simulink model "hdl_model_fixed"  (R2024a)
settings: Solver=FixedStepDiscrete  StartTime=0.0  StopTime=SIM_TIME  RelTol=1e-3
model workspace (MAT data in the model file):
  HDLVAXIManagerConfig = hdlverifier.internal.AXIMaster.ConfigParams
undefined symbols (not defined in the file or in its folder): BUFFER_LEN, SAMPLING_FREQ, signal_1
libraries: hdlsllib x4, simulink x1, dspsrcs4 x1, simulink_extras x1, dsphdlxfrm2 x1
settings Model: DataTypeOverride=Off  SimulationMode=accelerator  Creator=Jan Rosa  LastModifiedBy=Jan Rosa
settings OptimizationCC: BlockReduction=off  ConditionallyExecuteInputs=off  DefaultParameterBehavior=Inlined  InheritOutputTypeSmallerThanSingle=on
settings DebuggingCC: SignalRangeChecking=warning  AlgebraicLoopMsg=error  SolverPrmCheckMsg=warning  SingleTaskRateTransMsg=error  UnderSpecifiedDataTypeMsg=warning  UnconnectedInputMsg=error  UnconnectedOutputMsg=error  UnconnectedLineMsg=error  ModelReferenceVersionMismatchMessage=warning  ModelReferenceIOMismatchMessage=warning  ModelReferenceNoExplicitFinalValueMsg=warning  StateNameClashWarn=warning
settings HardwareCC: ProdBitPerPointer=32  ProdBitPerSizeT=32  ProdBitPerPtrDiffT=32  ProdLargestAtomicFloat=None  ProdIntDivRoundTo=Undefined  ProdEndianess=Unspecified  ProdWordSize=32  ProdHWDeviceType=ASIC/FPGA->ASIC/FPGA  TargetBitPerPointer=64  TargetBitPerSizeT=64  TargetBitPerPtrDiffT=64  TargetLongLongMode=on  TargetIntDivRoundTo=Zero  TargetEndianess=LittleEndian  TargetWordSize=64  TargetHWDeviceType=Custom Processor->MATLAB Host Computer  ProdEqTarget=off
settings ModelReferenceCC: EnableRefExpFcnMdlSchedulingChecks=on  EnableParallelModelReferenceBuilds=on

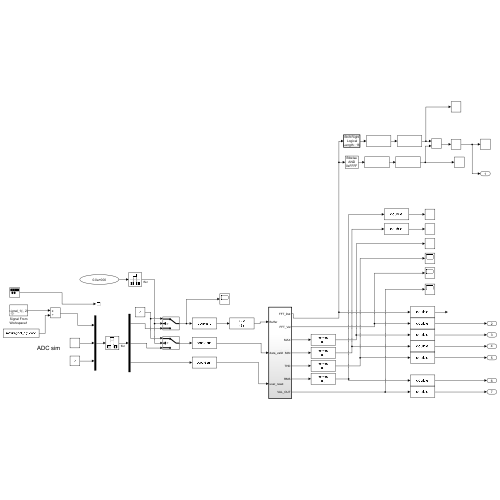
[thumbnail: Simulink's stored preview of the top-level diagram]
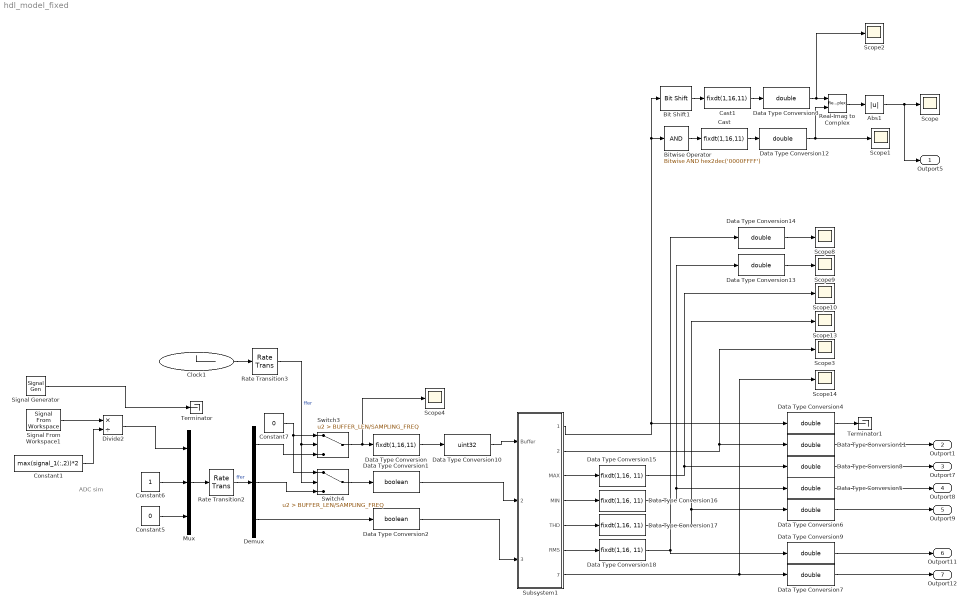
== system hdl_model_fixed ==
  note: ADC sim
  Abs1 : Abs  SaturateOnIntegerOverflow=off
  Bit Shift1 : hdlsllib/Logic and Bit Operations/Bit Shift  mode=Shift Right Logical  N=16
  Bitwise Operator : simulink/Logic and Bit Operations/Bitwise Operator  logicop=AND  UseBitMask=on  BitMask=hex2dec('0000FFFF')  BitMaskRealWorld=Stored Integer
  Cast : DataTypeConversion  OutDataTypeStr=fixdt(1,16,11)  ConvertRealWorld=Stored Integer (SI)  SaturateOnIntegerOverflow=off  RndMeth=Floor
  Cast1 : DataTypeConversion  OutDataTypeStr=fixdt(1,16,11)  ConvertRealWorld=Stored Integer (SI)  SaturateOnIntegerOverflow=off  RndMeth=Floor
  Clock1 : Clock
  Constant1 : Constant  Value=max(signal_1(:,2))*2
  Constant5 : Constant  Value=0
  Constant6 : Constant
  Constant7 : Constant  Value=0  SampleTime=1/SAMPLING_FREQ
  Data Type Conversion : DataTypeConversion  OutDataTypeStr=fixdt(1,16,11)  SaturateOnIntegerOverflow=off  RndMeth=Floor  LockScale=on
  Data Type Conversion1 : DataTypeConversion  OutDataTypeStr=boolean  SaturateOnIntegerOverflow=off  RndMeth=Floor  LockScale=on
  Data Type Conversion10 : DataTypeConversion  OutDataTypeStr=uint32  ConvertRealWorld=Stored Integer (SI)  SaturateOnIntegerOverflow=off  RndMeth=Floor
  Data Type Conversion{3..9,11..14} (11 alike) : DataTypeConversion  OutDataTypeStr=double  SaturateOnIntegerOverflow=off  RndMeth=Floor
  Data Type Conversion{15..18} (4 alike) : DataTypeConversion  OutDataTypeStr=fixdt(1,16, 11)  ConvertRealWorld=Stored Integer (SI)  SaturateOnIntegerOverflow=off  RndMeth=Floor
  Data Type Conversion2 : DataTypeConversion  OutDataTypeStr=boolean  SaturateOnIntegerOverflow=off  RndMeth=Floor  LockScale=on
  Demux : Demux  Outputs=3
  Divide2 : Product  Inputs=*/
  Mux : Mux  Inputs=3
  Rate Transition2 : RateTransition  Integrity=off  Deterministic=off  OutPortSampleTime=1/SAMPLING_FREQ
  Rate Transition3 : RateTransition  Integrity=off  Deterministic=off  OutPortSampleTime=1/SAMPLING_FREQ
  Real-Imag to Complex : RealImagToComplex
  Scope{,1..4,8..10,13..14} (10 alike) : Scope
  Signal Generator : SignalGenerator  WaveForm=square  Amplitude=1/2.001  Frequency=SAMPLING_FREQ/(16*16)
  Signal From Workspace1 : dspsrcs4/Signal From Workspace  X=signal_1(:, 2)  Ts=1.28/SAMPLING_FREQ  nsamps=1  OutputAfterFinalValue=Cyclic repetition  ignoreOrWarnInputAndFrameLengths=off  OutputFrames=off
  Subsystem1 : Subsystem  TreatAsAtomicUnit=on
  Switch3 : Switch  Criteria=u2 > Threshold  Threshold=BUFFER_LEN/SAMPLING_FREQ  SaturateOnIntegerOverflow=off  InputSameDT=off
  Switch4 : Switch  Criteria=u2 > Threshold  Threshold=BUFFER_LEN/SAMPLING_FREQ  SaturateOnIntegerOverflow=off  InputSameDT=off
  Terminator : Terminator
  Terminator1 : Terminator
  Outport5 : Outport
  Outport1 : Outport  Port=2
  Outport7 : Outport  Port=3
  Outport8 : Outport  Port=4
  Outport9 : Outport  Port=5
  Outport11 : Outport  Port=6
  Outport12 : Outport  Port=7
  wires:
  Subsystem1/1(FFT_Dat) -> Data Type Conversion4/1, Bitwise Operator/1, Bit Shift1/1
  Constant7/1 -> Switch4/1, Switch3/1
  Rate Transition3/1 -> Switch4/2, Switch3/2  "ffer"
  Subsystem1/7(VAL_OUT) -> Data Type Conversion7/1, Scope14/1
  Subsystem1/3(MAX) -> Data Type Conversion15/1
  Demux/2 -> Switch4/3
  Clock1/1 -> Rate Transition3/1
  Demux/3 -> Data Type Conversion2/1
  Subsystem1/5(THD) -> Data Type Conversion17/1
  Switch3/1 -> Scope4/1, Data Type Conversion/1
  Demux/1 -> Switch3/3
  Mux/1 -> Rate Transition2/1
  Subsystem1/4(MIN) -> Data Type Conversion16/1
  Abs1/1 -> Outport5/1, Scope/1
  Rate Transition2/1 -> Demux/1  "ffer"
  Constant5/1 -> Mux/3
  Signal From Workspace1/1 -> Divide2/1
  Constant6/1 -> Mux/2
  Constant1/1 -> Divide2/2
  Subsystem1/6(RMS) -> Data Type Conversion18/1
  Data Type Conversion8/1 -> Outport7/1
  Data Type Conversion5/1 -> Outport8/1
  Data Type Conversion6/1 -> Outport9/1
  Data Type Conversion7/1 -> Outport12/1
  Data Type Conversion9/1 -> Outport11/1
  Data Type Conversion11/1 -> Outport1/1
  Data Type Conversion3/1 -> Scope2/1, Real-Imag to Complex/1
  Real-Imag to Complex/1 -> Abs1/1
  Bit Shift1/1 -> Cast1/1
  Bitwise Operator/1 -> Cast/1
  Data Type Conversion12/1 -> Scope1/1, Real-Imag to Complex/2
  Cast/1 -> Data Type Conversion12/1
  Cast1/1 -> Data Type Conversion3/1
  Data Type Conversion14/1 -> Scope8/1
  Data Type Conversion13/1 -> Scope9/1
  Switch4/1 -> Data Type Conversion1/1
  Data Type Conversion2/1 -> Subsystem1/3(user_reset)
  Data Type Conversion1/1 -> Subsystem1/2(data_valid)
  Data Type Conversion/1 -> Data Type Conversion10/1
  Subsystem1/2(FFT_Val) -> Scope3/1, Data Type Conversion11/1
  Data Type Conversion10/1 -> Subsystem1/1(Buffer)
  Data Type Conversion15/1 -> Data Type Conversion8/1, Scope10/1
  Data Type Conversion16/1 -> Data Type Conversion5/1, Data Type Conversion13/1
  Data Type Conversion17/1 -> Data Type Conversion6/1, Scope13/1
  Data Type Conversion18/1 -> Data Type Conversion9/1, Data Type Conversion14/1
  Data Type Conversion4/1 -> Terminator1/1
  Signal Generator/1 -> Terminator/1
  Divide2/1 -> Mux/1

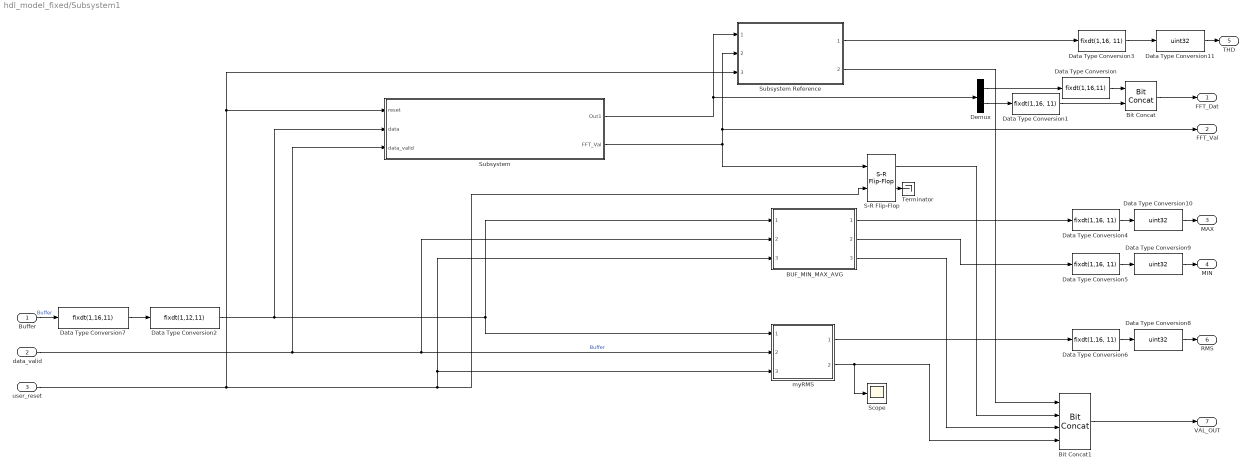
== system hdl_model_fixed/Subsystem1 ==
  Buffer : Inport  OutDataTypeStr=uint32
  data_valid : Inport  Port=2
  user_reset : Inport  Port=3
  BUF_MIN_MAX_AVG : Subsystem  TreatAsAtomicUnit=on  ReferencedSubsystem=BUF_MIN_MAX_AVG_fixed
  Bit Concat : hdlsllib/Logic and Bit Operations/Bit Concat  numInputs=2
  Bit Concat1 : hdlsllib/Logic and Bit Operations/Bit Concat  numInputs=4
  Data Type Conversion : DataTypeConversion  OutDataTypeStr=fixdt(1,16,11)  SaturateOnIntegerOverflow=off  RndMeth=Floor
  Data Type Conversion{1,3..6} (5 alike) : DataTypeConversion  OutDataTypeStr=fixdt(1,16, 11)  SaturateOnIntegerOverflow=off  RndMeth=Floor
  Data Type Conversion{8..11} (4 alike) : DataTypeConversion  OutDataTypeStr=uint32  ConvertRealWorld=Stored Integer (SI)  SaturateOnIntegerOverflow=off  RndMeth=Floor
  Data Type Conversion2 : DataTypeConversion  OutDataTypeStr=fixdt(1,12,11)  SaturateOnIntegerOverflow=off  RndMeth=Floor
  Data Type Conversion7 : DataTypeConversion  OutDataTypeStr=fixdt(1,16,11)  ConvertRealWorld=Stored Integer (SI)  SaturateOnIntegerOverflow=off  RndMeth=Floor
  Demux : Demux  Outputs=2
  S-R Flip-Flop : simulink_extras/Flip Flops/S-R Flip-Flop  initial_condition=0
  Scope : Scope
  Subsystem : Subsystem  TreatAsAtomicUnit=on
  Subsystem Reference : Subsystem  TreatAsAtomicUnit=on  ReferencedSubsystem=myTHD_fixed
  Terminator : Terminator
  myRMS : Subsystem  TreatAsAtomicUnit=on  ReferencedSubsystem=myRMS_fixed
  FFT_Dat : Outport
  FFT_Val : Outport  Port=2
  MAX : Outport  Port=3
  MIN : Outport  Port=4
  THD : Outport  Port=5
  RMS : Outport  Port=6
  VAL_OUT : Outport  Port=7
  wires:
  BUF_MIN_MAX_AVG/3 -> Bit Concat1/3
  myRMS/2 -> Scope/1, Bit Concat1/4
  Buffer/1 -> Data Type Conversion7/1  "Buffer"
  data_valid/1 -> Subsystem/3(data_valid), myRMS/2, BUF_MIN_MAX_AVG/2  "Buffer"
  Subsystem Reference/2 -> Bit Concat1/1
  S-R Flip-Flop/1 -> Bit Concat1/2
  S-R Flip-Flop/2 -> Terminator/1
  Subsystem/2(FFT_Val) -> S-R Flip-Flop/1, FFT_Val/1, Subsystem Reference/2
  BUF_MIN_MAX_AVG/1 -> Data Type Conversion4/1
  BUF_MIN_MAX_AVG/2 -> Data Type Conversion5/1
  myRMS/1 -> Data Type Conversion6/1
  Bit Concat1/1 -> VAL_OUT/1
  Subsystem Reference/1 -> Data Type Conversion3/1
  Bit Concat/1 -> FFT_Dat/1
  Data Type Conversion3/1 -> Data Type Conversion11/1
  Data Type Conversion4/1 -> Data Type Conversion10/1
  Data Type Conversion5/1 -> Data Type Conversion9/1
  Data Type Conversion6/1 -> Data Type Conversion8/1
  Data Type Conversion2/1 -> Subsystem/2(data), BUF_MIN_MAX_AVG/1, myRMS/1
  user_reset/1 -> Subsystem Reference/3, Subsystem/1(reset), BUF_MIN_MAX_AVG/3, myRMS/3, S-R Flip-Flop/2
  Subsystem/1(Out1) -> Subsystem Reference/1, Demux/1
  Demux/2 -> Data Type Conversion1/1
  Demux/1 -> Data Type Conversion/1
  Data Type Conversion/1 -> Bit Concat/1
  Data Type Conversion1/1 -> Bit Concat/2
  Data Type Conversion7/1 -> Data Type Conversion2/1
  Data Type Conversion8/1 -> RMS/1
  Data Type Conversion9/1 -> MIN/1
  Data Type Conversion10/1 -> MAX/1
  Data Type Conversion11/1 -> THD/1

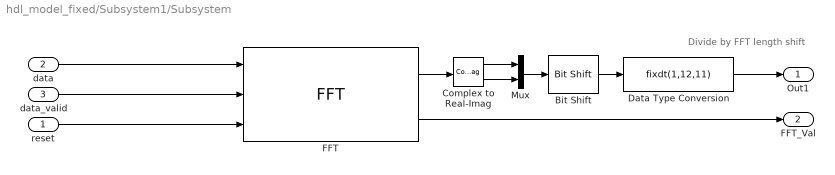
== system hdl_model_fixed/Subsystem1/Subsystem ==
  note: Divide by FFT length shift
  reset : Inport
  data : Inport  Port=2
  data_valid : Inport  Port=3
  Bit Shift : hdlsllib/Logic and Bit Operations/Bit Shift  mode=Shift Right Arithmetic  N=log2(BUFFER_LEN)
  Complex to Real-Imag : ComplexToRealImag
  Data Type Conversion : DataTypeConversion  OutDataTypeStr=fixdt(1,12,11)  SaturateOnIntegerOverflow=off  RndMeth=Floor
  FFT : dsphdlxfrm2/FFT  Architecture=Streaming Radix 2^2  FFTLengthSource=Property  FFTLength=BUFFER_LEN  FFTLengthMax=1024  ComplexMultiplication=Use 4 multipliers and 2 adders  BitReversedOutput=off  BitReversedInput=off  Normalize=off  SimulateUsing=Code generation  RoundingMethod=Floor  ResetInputPort=on  StartOutputPort=off  EndOutputPort=off
  Mux : Mux  Inputs=2
  Out1 : Outport
  FFT_Val : Outport  Port=2
  wires:
  Bit Shift/1 -> Data Type Conversion/1
  Complex to Real-Imag/1 -> Mux/1
  data/1 -> FFT/1
  reset/1 -> FFT/3
  data_valid/1 -> FFT/2
  Mux/1 -> Bit Shift/1
  Complex to Real-Imag/2 -> Mux/2
  FFT/1 -> Complex to Real-Imag/1
  Data Type Conversion/1 -> Out1/1
  FFT/2 -> FFT_Val/1
